simulink model "pll01"  (Simulink 8.1)
settings: Solver=ode45  StartTime=0.0  StopTime=10  MaxStep=0.0001  RelTol=1e-3
libraries: commsynccomp2 x1, simulink x1
settings Model: Creator=my88899  LastModifiedBy=my88899
settings DataIOCC: SignalLoggingSaveFormat=Dataset
settings OptimizationCC: ExpressionDepthLimit=128
settings DebuggingCC: FcnCallInpInsideContextMsg=EnableAllAsError
settings GRTTargetCC: CombineOutputUpdateFcns=on  GRTInterface=off

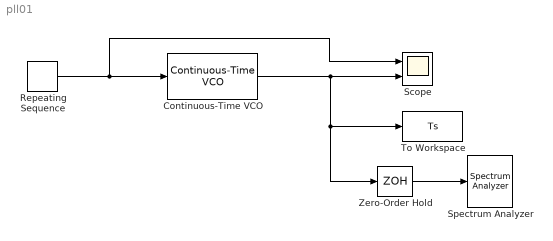
== system pll01 ==
  Continuous-Time VCO : commsynccomp2/Continuous-Time VCO  Ac=5  Fc=100  Kc=100  Ph=0
  Repeating Sequence : simulink/Sources/Repeating Sequence  rep_seq_t=[0 1]  rep_seq_y=[0 5]
  Scope : Scope  NumInputPorts=2
      settings: TimeRange=0.1038961038961048  YMin=5.645~-5  YMax=5.7~5  MaxDataPoints=100000
  Spectrum Analyzer : SpectrumAnalyzer
      settings: CopyFcn=scopeextensions.ScopeBlock.callback(gcbh, 'onBlockCopy', gcbh);  DeleteFcn=scopeextensions.ScopeBlock.callback(gcbh, 'onBlockDelete');  PreSaveFcn=scopeextensions.ScopeBlock.callback(gcbh, 'onModelSave');  NameChangeFcn=scopeextensions.ScopeBlock.callback(gcbh, 'onBlockRename');  CloseFcn=scopeextensions.ScopeBlock.callback(gcbh, 'onBlockClose');  PreDeleteFcn=scopeextensions.ScopeBlock.callback(gcbh, 'onBlockPreDelete');
  To Workspace : ToWorkspace  VariableName=Ts  SampleTime=-1  SaveFormat=Timeseries
  Zero-Order Hold : ZeroOrderHold  SampleTime=0.01
  wires:
  Repeating Sequence/1 -> Scope/1, Continuous-Time VCO/1
  Continuous-Time VCO/1 -> To Workspace/1, Zero-Order Hold/1, Scope/2
  Zero-Order Hold/1 -> Spectrum Analyzer/1
